simulink model "Sum"  (R2020a)
settings: Solver=VariableStepAuto  StartTime=0.0  StopTime=10.0  RelTol=1e-3
settings Model: Creator=royde  LastModifiedBy=royde

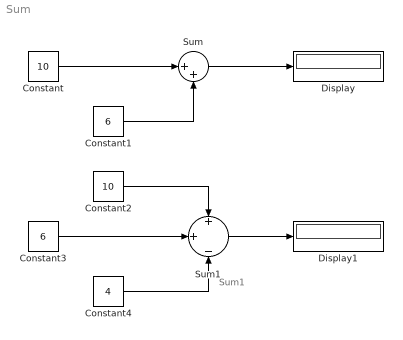
== system Sum ==
  note: Sum1
  Constant : Constant  Value=10
  Constant1 : Constant  Value=6
  Constant2 : Constant  Value=10
  Constant3 : Constant  Value=6
  Constant4 : Constant  Value=4
  Display : Display
  Display1 : Display
  Sum : Sum  Inputs=|++
  Sum1 : Sum  Inputs=+|+|-
  wires:
  Constant/1 -> Sum/1
  Constant1/1 -> Sum/2
  Sum/1 -> Display/1
  Sum1/1 -> Display1/1
  Constant3/1 -> Sum1/2
  Constant2/1 -> Sum1/1
  Constant4/1 -> Sum1/3
